simulink model "Tanques_desacoplados"  (R2021b)
settings: Solver=FixedStepAuto  StartTime=0.0  StopTime=120  RelTol=1e-3  AbsTol=1e-3  EnableMultiTasking=on
libraries: sh_lib x5, fl_lib x4, nesl_utility x4, slrealtimeseriallib x2, raspberrypiCommlib x2
settings Model: Creator=Pc melhor q do euler  LastModifiedBy=Pc melhor q do euler
settings SolverCC: AutoScaleAbsTol=off  AlgebraicLoopSolver=TrustRegion  PositivePriorityOrder=on
settings OptimizationCC: EnhancedBackFolding=on  PassReuseOutputArgsAs=Individual arguments  ZeroExternalMemoryAtStartup=off  ZeroInternalMemoryAtStartup=off  MaxStackSize=64  OptimizeBlockOrder=speed  DifferentSizesBufferReuse=on  OptimizationCustomize=off  EfficientTunableParamExpr=on
settings DebuggingCC: ParameterTunabilityLossMsg=error  SymbolicDimsDataTypeCodeGenerationDiagnostic=none  SFMachineParentedDataDiag=warning
settings HardwareCC: ProdBitPerPointer=32  ProdBitPerSizeT=32  ProdBitPerPtrDiffT=32  ProdLargestAtomicInteger=Long  ProdLargestAtomicFloat=Double  ProdWordSize=32  ProdLongLongMode=on  ProdHWDeviceType=ARM Compatible->ARM Cortex
settings SFSimCC: CustomCodeUndefinedFunction=UseInterfaceOnly
settings RTWCC: Description=Embedded Coder  SystemTargetFile=ert.tlc  HardwareBoard=Raspberry Pi  TLCOptions="-aInlineSetEventsForThisBaseRateFcn=TLC_FALSE -aSuppressMultiTaskScheduler=TLC_FALSE  -aRateBasedStepFcn=0"  TemplateMakefile=ert_default_tmf  Toolchain=GNU GCC Embedded Linux  BuildConfiguration=Faster Runs
settings CodeAppCC: ForceParamTrailComments=on  IgnoreCustomStorageClasses=off  OperatorAnnotations=on  SimulinkDataObjDesc=on  SFDataObjDesc=on  InsertBlockDesc=on
settings ERTTargetCC: SupportVariableSizeSignals=on  ExtModeTransport=2  ExtModeStaticAlloc=on  ExtModeMexFile=ext_xcp  ExtModeIntrfLevel=Level2 - Open
settings SimscapeCC: SimscapeLogType=all  SimscapeLogSimulationStatistics=on  SimscapeLogDataHistory=10000

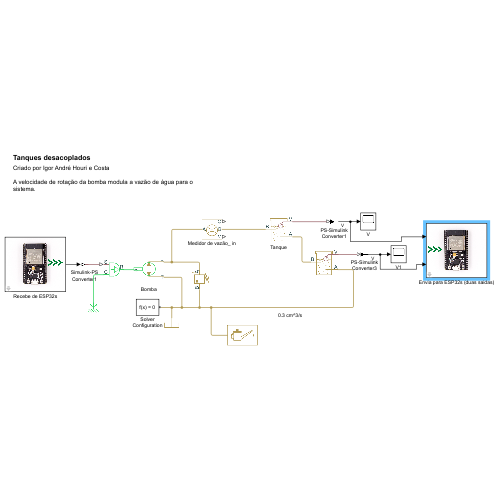
[thumbnail: Simulink's stored preview of the top-level diagram]
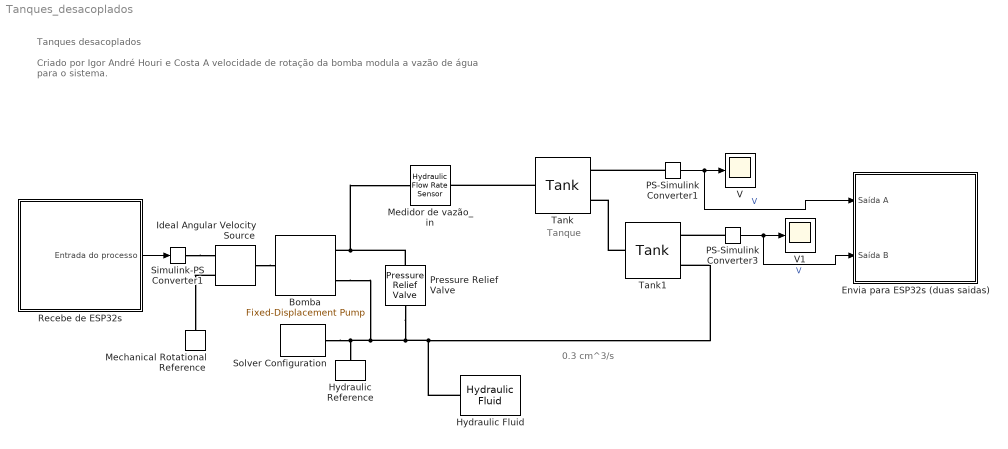
== system Tanques_desacoplados ==
  note: 0.3 cm^3/s
  note: Tanque
  note: Tanques desacoplados
  note: Criado por Igor André Houri e Costa
      |
      | A velocidade de rotação da bomba modula a vazão de água para o sistema.
  Bomba : sh_lib/Pumps and Motors/Fixed-Displacement Pump  D=5 cm^3/rev  loss_spec=1  w_nominal=188 rad/s  pr_nominal=100e5 Pa  visc_nominal=1.003 cSt  dens_nominal=1000 kg/m^3  efficiency_vol=0.92  no_load_torque=0.05 N*m  torque_pressure_coeff=0.6e-6 N*m/Pa  p_diff_eff_TLU=[100000, 1000000, 2000000] Pa  omega_eff_TLU=[25, 50, 100, 200, 300, 400] rad/s  vol_eff_TLU=[.816, .908, .954, .977, .981, .984; .325, .663, .831, .916, .925, .946; .137, .568, .78, .892, .893, .91]  mech_eff_TLU=[.996, .996, .996, .996, .996, .996; .988, .989, .989, .989, .989, .99; .981, .981, .982, .982, .983, .984]  p_diff_loss_TLU=[100000, 1000000, 2000000] Pa  omega_loss_TLU=[25, 50, 100, 200, 300, 400] rad/s  vol_loss_TLU=[.023, .023, .023, .023, .0285, .032; .0844, .0842, .0845, .084, .1125, .108; .1079, .108, .11, .108, .1605, .18] * 1e-3 m^3/s  mech_loss_TLU=[.002, .002, .002, .002, .002, .002; .0607, .0556, .0556, .0556, .0556, .0505; .1937, .1937, .1833, .1833, .1729, .1626] N*m  pressure_threshold=1e5 Pa  omega_threshold=10 rad/s  quadrant_check=0  pressure_check=0  min_valid_pressure=0 Pa  vol_eff_min=1e-3  vol_eff_max=1  mech_eff_min=1e-3  mech_eff_max=1
      settings: SourceProductBaseCode=SH  InternalSimscapePortConfiguration="{\"Bottom\":[],\"Left\":[{\"id\":\"S\",\"label\":\"S\",\"type\":\"foundation.mechanical.rotational.rotational\"}],\"Right\":[{\"id\":\"P\",\"label\":\"P\",\"type\":\"foundation.hydraulic.hydraulic\"},{\"id\":\"T\",\"label\":\"T\",\"type\":\"foundation.hydraulic.hydraulic\"}],\"Top\":[]}"
  Envia para ESP32s (duas saidas) : Subsystem  mask{board=Pi 3 Model B, SCIModule_=/dev/ttyS0, Baudrate_=9600, SaidaMaximaA=25, SaidaMinimaA=0, SaidaMaximaB=10, SaidaMinimaB=0}
      mask prompts: board "Placa"; SCIModule_ "Port:"; Baudrate_ "Baudrate (in bits/s):"; SaidaMaximaA "Saída Máxima A"; SaidaMinimaA "Saida Mínima A"; SaidaMaximaB "Saída Máxima B"; SaidaMinimaB "Saída Mínima B"
      mask TypeOptions board: Serial Write/board
      mask TypeOptions SCIModule_: Serial Write/SCIModule_
      mask TypeOptions Baudrate_: Serial Write/Baudrate_
      mask TypeOptions SaidaMaximaA: Função Map (saídaA)/SaidaMaximaA
      mask TypeOptions SaidaMinimaA: Função Map (saídaA)/SaidaMinimaA
      mask TypeOptions SaidaMaximaB: Função Map (saídaB)/SaidaMaximaB
      mask TypeOptions SaidaMinimaB: Função Map (saídaB)/SaidaMinimaB
      mask Display: image('I:\PFC_Igor\plot figuras\figuras\Envia para ESP32s.png'); % Use "Edit Image" on toolstrip to change.
  Hydraulic Fluid : sh_lib/Hydraulic Utilities/Hydraulic Fluid  DataSource=1  SelFluid=24  SysTemp=60  TrapAir=0.005  ViscDerFactor=1  range_error=2
  Hydraulic Reference : fl_lib/Hydraulic/Hydraulic Elements/Hydraulic Reference
  Ideal Angular Velocity Source : fl_lib/Mechanical/Mechanical Sources/Ideal Angular Velocity Source
  Mechanical Rotational Reference : fl_lib/Mechanical/Rotational Elements/Mechanical Rotational Reference
  Medidor de vazão_ in : fl_lib/Hydraulic/Hydraulic Sensors/Hydraulic Flow Rate Sensor
  PS-Simulink Converter1 : nesl_utility/PS-Simulink Converter  PhysicalDomain=network_engine_domain  SubClassName=ps_output  LeftPortType=input  RightPortType=output  PseudoPeriodic=off  Frequencies=[]  Unit=l  AffineConversion=off
      settings: SourceProductBaseCode=PW,SS
  PS-Simulink Converter3 : nesl_utility/PS-Simulink Converter  PhysicalDomain=network_engine_domain  SubClassName=ps_output  LeftPortType=input  RightPortType=output  PseudoPeriodic=off  Frequencies=[]  Unit=l  AffineConversion=off
      settings: SourceProductBaseCode=PW,SS
  Pressure Relief Valve : sh_lib/Valves/Pressure Control Valves/Pressure Relief Valve  valve_area_spec=1  p_diff_TLU=[30.15e5 : 15e3 : 31.35e5] Pa  area_TLU=[1 : 1 : 9] .* 1e-5 m^2  area_max=1e-4 m^2  pres_set=50e5 Pa  reg_range=5e5 Pa  C_d=0.7  A_leak=1e-12 m^2  lam_spec=1  B_lam=0.999  Re_cr=12  dynamic=0  tau=0.1 s  area_init=1e-12 m^2
      settings: SourceProductBaseCode=SH  InternalSimscapePortConfiguration="{\"Bottom\":[],\"Left\":[{\"id\":\"A\",\"label\":\"A\",\"type\":\"foundation.hydraulic.hydraulic\"}],\"Right\":[{\"id\":\"B\",\"label\":\"B\",\"type\":\"foundation.hydraulic.hydraulic\"}],\"Top\":[]}"
  Recebe de ESP32s : Subsystem  mask(Recepção de mensagem Serial - ESP32s){board=Pi 3 Model B, SCIModule_=/dev/ttyS0, Baudrate_=115200, entrada_maxima=3, entrada_minima=0}
      mask prompts: SCIModule_ "Port:"; Baudrate_ "Baudrate (in bits/s):"; entrada_maxima "Entrada máxima do processo"; entrada_minima "Entrada mínima do processo"
      mask help: Este bloco recebe a mensagem serial enviada pelo ESP32s, decodifica-a e converte para a escala configurada; disponibilizando o resultado em sua saída. --Bloco criado por Igor Costa.
      mask TypeOptions board: Serial Read1/board
      mask TypeOptions SCIModule_: Serial Read1/SCIModule_
      mask TypeOptions Baudrate_: Serial Read1/Baudrate_
      mask TypeOptions entrada_maxima: Função Map (entrada)/entrada_maxima
      mask TypeOptions entrada_minima: Função Map (entrada)/entrada_minima
      mask Display: image('I:\PFC_Igor\plot figuras\figuras\Recebe de ESP32s.png'); % Use "Edit Image" on toolstrip to change.
  Simulink-PS Converter1 : nesl_utility/Simulink-PS Converter  PhysicalDomain=network_engine_domain  SubClassName=ps_input  LeftPortType=input  RightPortType=output  PseudoPeriodic=off  Frequencies=[]  NoiseDistribution=none  NoiseParameters=[]  Unit=rad/s  AffineConversion=off  FilteringAndDerivatives=provide  SimscapeFilterOrder=1  InputFilterTimeConstant=0.001  UdotUserProvided=0
      settings: SourceProductBaseCode=PW,SS
  Solver Configuration : nesl_utility/Solver Configuration  PhysicalDomain=network_engine_domain  SubClassName=solver  LeftPortType=input  RightPortType=generic  Tones=[]  Harmonics=[]  SimulateNoise=off  Profile=off  UseLocalSampling=off  EnableSwitchedLinearOptims=on  FrequencyDomain=off  UseCCode=off  RelTol=0.001  AbsTol=1e-06  MinStep=1e-09  ToWorkspace=off  RevertToSquareIcSolve=off  NumHomotopyIterations=100  PhasorMode=off  PhasorModeNumHarmonics=1  DoDC=off  ResidualTolerance=1e-09  UseLocalSolver=on  LocalSolverChoice=NE_BACKWARD_EULER_ADVANCER  LocalSolverSampleTime=0.001  DoFixedCost=on  MaxNonlinIter=3  MaxModeIter=2  ComputeImpulses=off  ImpulseIterations=2  LinearAlgebra=auto  EquationFormulation=NE_TIME_EF  DelaysMemoryBudget=1024  AutomaticFiltering=on  FilteringTimeConstant=0.001  PartitionStorageMethod=AS_NEEDED  PartitionMemoryBudget=1024  PartitionMethod=ROBUST
      settings: SourceProductBaseCode=PW,SS
  Tank : sh_lib/Low-Pressure Blocks/Tank  press=0 Pa  level_spec=1  tank_area=10 m^2  fluid_volume_tab=[0, .0028, .0065, .0114, .0176, .0252, .0344, .0436, .0512, .0574, .0623, .066, .0688, .0707, .072, .0727] m^3  fluid_level_tab=[0, .02, .04, .06, .08, .1, .12, .14, .16, .18, .2, .22, .24, .26, .28, .3] m  interp_method=1  extrap_method=1  pipe_diam=0.02 m  loss_coeff=1.2  g=9.80665 m/s^2  min_level=1e-3 m  fluid_level_check=0  volume_specify=on  volume_priority=High  volume=2 l  volume_nominal_specify=off  volume_nominal_unit=l  volume_nominal_value=1  level_specify=off  level_priority=None  level=1 m  level_nominal_specify=off  level_nominal_unit=m  level_nominal_value=1  pipe_diam_A=2 cm  loss_coeff_A=1.2  height_B=5 m  pipe_diam_B=3.56 m  loss_coeff_B=1.2  height_C=0.8 m  pipe_diam_C=0.02 m  loss_coeff_C=1.2
      settings: SourceProductBaseCode=SH  InternalSimscapePortConfiguration="{\"Bottom\":[],\"Left\":[{\"id\":\"B\",\"label\":\"B\",\"type\":\"foundation.hydraulic.hydraulic\"}],\"Right\":[{\"id\":\"V\",\"label\":\"V\",\"type\":\"output\"},{\"id\":\"A\",\"label\":\"A\",\"type\":\"foundation.hydraulic.hydraulic\"}],\"Top\":[]}"
  Tank1 : sh_lib/Low-Pressure Blocks/Tank  press=0 Pa  level_spec=1  tank_area=10 m^2  fluid_volume_tab=[0, .0028, .0065, .0114, .0176, .0252, .0344, .0436, .0512, .0574, .0623, .066, .0688, .0707, .072, .0727] m^3  fluid_level_tab=[0, .02, .04, .06, .08, .1, .12, .14, .16, .18, .2, .22, .24, .26, .28, .3] m  interp_method=1  extrap_method=1  pipe_diam=0.02 m  loss_coeff=1.2  g=9.80665 m/s^2  min_level=1e-3 m  fluid_level_check=0  volume_specify=on  volume_priority=High  volume=1 l  volume_nominal_specify=off  volume_nominal_unit=l  volume_nominal_value=1  level_specify=off  level_priority=None  level=1 m  level_nominal_specify=off  level_nominal_unit=m  level_nominal_value=1  pipe_diam_A=2 cm  loss_coeff_A=1.2  height_B=5 m  pipe_diam_B=3.56 m  loss_coeff_B=1.2  height_C=0.8 m  pipe_diam_C=0.02 m  loss_coeff_C=1.2
      settings: SourceProductBaseCode=SH  InternalSimscapePortConfiguration="{\"Bottom\":[],\"Left\":[{\"id\":\"B\",\"label\":\"B\",\"type\":\"foundation.hydraulic.hydraulic\"}],\"Right\":[{\"id\":\"V\",\"label\":\"V\",\"type\":\"output\"},{\"id\":\"A\",\"label\":\"A\",\"type\":\"foundation.hydraulic.hydraulic\"}],\"Top\":[]}"
  V : Scope
  V1 : Scope
  wires:
  PS-Simulink Converter1/1 -> Envia para ESP32s (duas saidas)/1(Saída A), V/1  "V"
  Recebe de ESP32s/1(Entrada do processo) -> Simulink-PS Converter1/1
  PS-Simulink Converter3/1 -> Envia para ESP32s (duas saidas)/2(Saída B), V1/1  "V"
  connections:
  Pressure Relief Valve/LConn1 -- Medidor de vazão_ in/LConn1 -- Bomba/RConn1
  Tank/LConn1 -- Medidor de vazão_ in/RConn2
  PS-Simulink Converter1/LConn1 -- Tank/RConn1
  Ideal Angular Velocity Source/LConn1 -- Bomba/LConn1
  Ideal Angular Velocity Source/RConn2 -- Mechanical Rotational Reference/LConn1
  Simulink-PS Converter1/RConn1 -- Ideal Angular Velocity Source/RConn1
  Tank1/LConn1 -- Tank/RConn2
  Hydraulic Fluid/RConn1 -- Tank1/RConn2 -- Solver Configuration/RConn1 -- Hydraulic Reference/LConn1 -- Bomba/RConn2 -- Pressure Relief Valve/RConn1
  PS-Simulink Converter3/LConn1 -- Tank1/RConn1

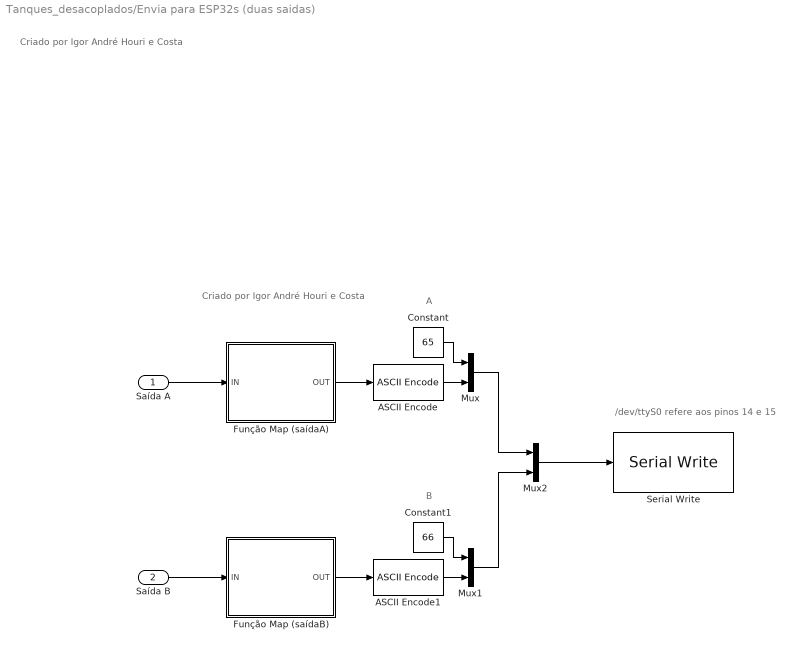
== system Tanques_desacoplados/Envia para ESP32s (duas saidas) ==
  note: B
  note: A
  note: /dev/ttyS0 refere aos pinos 14 e 15
  note: Criado por Igor André Houri e Costa
  note: Criado por Igor André Houri e Costa
  Saída A : Inport
  Saída B : Inport  Port=2
  ASCII Encode : slrealtimeseriallib/ASCII Encode  format=%d\r  nvars=1  maxlength=32  vartypes={ 'double' }
      settings: SourceProductBaseCode=XP
  ASCII Encode1 : slrealtimeseriallib/ASCII Encode  format=%d\r  nvars=1  maxlength=32  vartypes={ 'double' }
      settings: SourceProductBaseCode=XP
  Constant : Constant  Value=65  OutDataTypeStr=uint8
  Constant1 : Constant  Value=66  OutDataTypeStr=uint8
  Função Map (saídaA) : Subsystem  mask{SaidaMaximaA=SaidaMaximaA, SaidaMinimaA=SaidaMinimaA}
      mask prompts: SaidaMaximaA "Saída Máxima A"; SaidaMinimaA "Saida Mínima A"
      mask TypeOptions SaidaMaximaA: Saida_maximaA/Value
      mask TypeOptions SaidaMinimaA: Saida_minimaA/Value
  Função Map (saídaB) : Subsystem  mask{SaidaMaximaB=SaidaMaximaB, SaidaMinimaB=SaidaMinimaB}
      mask prompts: SaidaMaximaB "Saída Máxima B"; SaidaMinimaB "Saída Mínima B"
      mask TypeOptions SaidaMaximaB: Saida_maximaB/Value
      mask TypeOptions SaidaMinimaB: Saida_minimaB/Value
  Mux : Mux  Inputs=2
  Mux1 : Mux  Inputs=2
  Mux2 : Mux  Inputs=2
  Serial Write : raspberrypiCommlib/Serial Write  board=Pi 3 Model B  SCIModule_=/dev/ttyS0  Baudrate_=9600  Parity=None  StopBits_=1  HardwareFlowControl=None  ByteOrder=LittleEndian  OutputStatus=off  blockPlatform=RaspberryPi
      settings: SourceProductBaseCode=RASPPI
  wires:
  Função Map (saídaA)/1(OUT) -> ASCII Encode/1
  Saída A/1 -> Função Map (saídaA)/1(IN)
  Saída B/1 -> Função Map (saídaB)/1(IN)
  Função Map (saídaB)/1(OUT) -> ASCII Encode1/1
  ASCII Encode/1 -> Mux/2
  Constant/1 -> Mux/1
  ASCII Encode1/1 -> Mux1/2
  Constant1/1 -> Mux1/1
  Mux1/1 -> Mux2/2
  Mux/1 -> Mux2/1
  Mux2/1 -> Serial Write/1

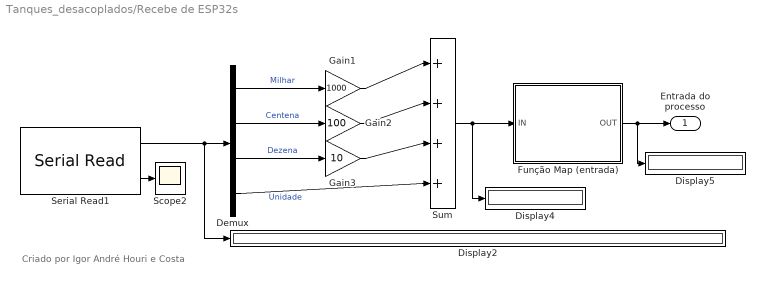
== system Tanques_desacoplados/Recebe de ESP32s ==
  note: Criado por Igor André Houri e Costa
  Demux : Demux
  Display2 : Display
  Display4 : Display
  Display5 : Display
  Função Map (entrada) : Subsystem  mask(Função Map - entrada){entrada_maxima=entrada_maxima, entrada_minima=entrada_minima}
      mask prompts: entrada_maxima "Entrada máxima do processo"; entrada_minima "Entrada mínima do processo"
      mask help: Este bloco mapeia um número de uma escala (range) da escala necessária para decodificação da entrada do processo recebida ESP32s (0 a 4095), passando-o para a escala dos valores do processo. A função implementada é (x - 0) * (x_max - x_min) / (4095 - 0), sendo "x" o valor do número a ser mapeado, "x_min" o menor valor possível para x e "x_max" o maior valor possível para x. --Bloco criado por Igor Costa.
      mask TypeOptions entrada_maxima: Entrada_maxima/Value
      mask TypeOptions entrada_minima: Entrada_minima/Value
  Gain1 : Gain  Gain=1000
  Gain2 : Gain  Gain=100
  Gain3 : Gain  Gain=10
  Scope2 : Scope
  Serial Read1 : raspberrypiCommlib/Serial Read  board=Pi 3 Model B  SCIModule_=/dev/ttyS0  Baudrate_=115200  Parity=None  StopBits_=1  HardwareFlowControl=None  ByteOrder=LittleEndian  DataLength=4  DataType=uint8  OutputStatus=on  SampleTime=0.1  blockPlatform=RaspberryPi
      settings: SourceProductBaseCode=RASPPI
  Sum : Sum  Inputs=|++++
  Entrada do processo : Outport
  wires:
  Demux/3 -> Gain3/1  "Dezena"
  Demux/4 -> Sum/4  "Unidade"
  Demux/2 -> Gain2/1  "Centena"
  Serial Read1/2 -> Scope2/1
  Demux/1 -> Gain1/1  "Milhar"
  Sum/1 -> Display4/1, Função Map (entrada)/1(IN)
  Gain1/1 -> Sum/1
  Gain2/1 -> Sum/2
  Serial Read1/1 -> Display2/1, Demux/1
  Gain3/1 -> Sum/3
  Função Map (entrada)/1(OUT) -> Display5/1, Entrada do processo/1

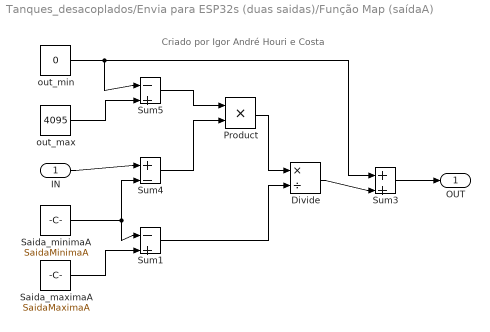
== system Tanques_desacoplados/Envia para ESP32s (duas saidas)/Função Map (saídaA) ==
  note: Criado por Igor André Houri e Costa
  IN : Inport
  Divide : Product  Inputs=*/
  Product : Product
  Saida_maximaA : Constant  Value=SaidaMaximaA
  Saida_minimaA : Constant  Value=SaidaMinimaA
  Sum1 : Sum  Inputs=|-+
  Sum3 : Sum  Inputs=++|
  Sum4 : Sum  Inputs=|+-
  Sum5 : Sum  Inputs=|-+
  out_max : Constant  Value=4095
  out_min : Constant  Value=0
  OUT : Outport
  wires:
  Sum5/1 -> Product/1
  out_max/1 -> Sum5/2
  Sum1/1 -> Divide/2
  Saida_minimaA/1 -> Sum4/2, Sum1/1
  IN/1 -> Sum4/1
  out_min/1 -> Sum3/1, Sum5/1
  Divide/1 -> Sum3/2
  Sum4/1 -> Product/2
  Product/1 -> Divide/1
  Sum3/1 -> OUT/1
  Saida_maximaA/1 -> Sum1/2

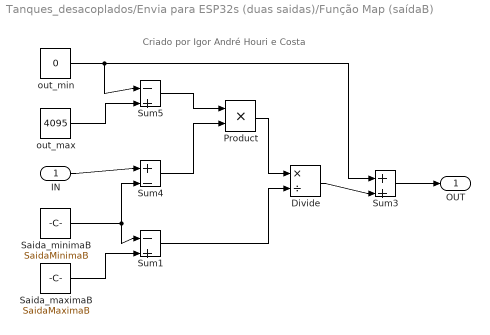
== system Tanques_desacoplados/Envia para ESP32s (duas saidas)/Função Map (saídaB) ==
  note: Criado por Igor André Houri e Costa
  IN : Inport
  Divide : Product  Inputs=*/
  Product : Product
  Saida_maximaB : Constant  Value=SaidaMaximaB
  Saida_minimaB : Constant  Value=SaidaMinimaB
  Sum1 : Sum  Inputs=|-+
  Sum3 : Sum  Inputs=++|
  Sum4 : Sum  Inputs=|+-
  Sum5 : Sum  Inputs=|-+
  out_max : Constant  Value=4095
  out_min : Constant  Value=0
  OUT : Outport
  wires:
  Sum5/1 -> Product/1
  out_max/1 -> Sum5/2
  Sum1/1 -> Divide/2
  Saida_minimaB/1 -> Sum4/2, Sum1/1
  IN/1 -> Sum4/1
  out_min/1 -> Sum3/1, Sum5/1
  Divide/1 -> Sum3/2
  Sum4/1 -> Product/2
  Product/1 -> Divide/1
  Sum3/1 -> OUT/1
  Saida_maximaB/1 -> Sum1/2

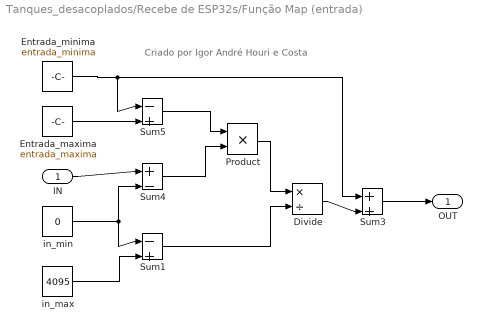
== system Tanques_desacoplados/Recebe de ESP32s/Função Map (entrada) ==
  note: Criado por Igor André Houri e Costa
  IN : Inport
  Divide : Product  Inputs=*/
  Entrada_maxima : Constant  Value=entrada_maxima
  Entrada_minima : Constant  Value=entrada_minima
  Product : Product
  Sum1 : Sum  Inputs=|-+
  Sum3 : Sum  Inputs=++|
  Sum4 : Sum  Inputs=|+-
  Sum5 : Sum  Inputs=|-+
  in_max : Constant  Value=4095
  in_min : Constant  Value=0
  OUT : Outport
  wires:
  Sum5/1 -> Product/1
  Sum1/1 -> Divide/2
  IN/1 -> Sum4/1
  Entrada_minima/1 -> Sum3/1, Sum5/1
  Divide/1 -> Sum3/2
  Sum4/1 -> Product/2
  Product/1 -> Divide/1
  Sum3/1 -> OUT/1
  in_max/1 -> Sum1/2
  in_min/1 -> Sum1/1, Sum4/2
  Entrada_maxima/1 -> Sum5/2
